simulink model "uncontrolled_simulink"  (R2020b)
settings: Solver=ode15s  StartTime=0.0  StopTime=T  MaxStep=0.01  RelTol=1e-3  EnableMultiTasking=on
values from neighbouring files (symbols this model uses):
  F_ee = zeros(6,1)    [sim_uncontrolled_simulink.m]
  g = [0 -g0 0]'    [sim_uncontrolled_simulink.m]
  info = struct('n_joints', n_joints,                'S', S,                'M_bi', M_bi,                'Inertia', Inertia,                'mass', mass,                'inertial_disp', inertial_disp)    [sim_uncontrolled_simulink.m]
  q_0 = [d0_0 alfa_0 beta_0]    [sim_uncontrolled_simulink.m]
  static_friction = [fs0 fs1 fs2]    [sim_uncontrolled_simulink.m]
  viscous_friction = [fv0 fv1 fv2]    [sim_uncontrolled_simulink.m]
settings Model: Creator=giank  LastModifiedBy=giank
settings DataIOCC: LimitDataPoints=on  MaxDataPoints=10000
settings OptimizationCC: LifeSpan=inf
settings DebuggingCC: AllowSymbolicDim=off  SFUnexpectedBacktrackingDiag=warning  SFNoUnconditionalDefaultTransitionDiag=warning  SFExecutionAtInitializationDiag=none  UnderSpecifiedDimensionMsg=warning  ArithmeticOperatorsInVariantConditions=warning
settings SFSimCC: SimUseLocalCustomCode=off  CustomCodeUndefinedFunction=UseInterfaceOnly
settings RTWCC: RTWUseLocalCustomCode=off
settings CodeAppCC: StateflowObjectComments=on
settings GRTTargetCC: TargetLangStandard=C89/C90 (ANSI)
settings ConfigComp: CovMetricSettings=dw  CovSaveCumulativeToWorkspaceVar=on  CovSaveSingleToWorkspaceVar=on  CovExternalEMLEnable=off  CovSFcnEnable=off
settings SimscapeCC: SimscapeLogType=all  SimscapeLogSimulationStatistics=on  SimscapeLogDataHistory=10000

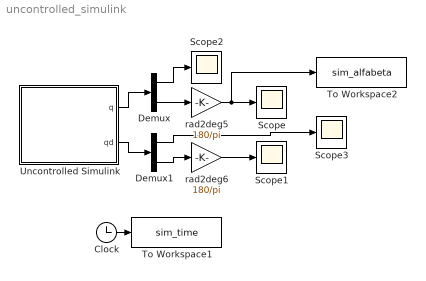
== system uncontrolled_simulink ==
  Clock : Clock
  Demux : Demux  Outputs=[1 2]
  Demux1 : Demux  Outputs=[1 2]
  Scope{,1..3} (4 alike) : Scope
  To Workspace1 : ToWorkspace  VariableName=sim_time  SaveFormat=Timeseries  SampleTime=-1
  To Workspace2 : ToWorkspace  VariableName=sim_alfabeta  SaveFormat=Timeseries  SampleTime=-1
  Uncontrolled Simulink : Subsystem
  rad2deg5 : Gain  Gain=180/pi
  rad2deg6 : Gain  Gain=180/pi
  wires:
  Clock/1 -> To Workspace1/1
  rad2deg6/1 -> Scope1/1
  rad2deg5/1 -> To Workspace2/1, Scope/1
  Demux/2 -> rad2deg5/1
  Uncontrolled Simulink/1(q) -> Demux/1
  Uncontrolled Simulink/2(qd) -> Demux1/1
  Demux1/2 -> rad2deg6/1
  Demux/1 -> Scope2/1
  Demux1/1 -> Scope3/1

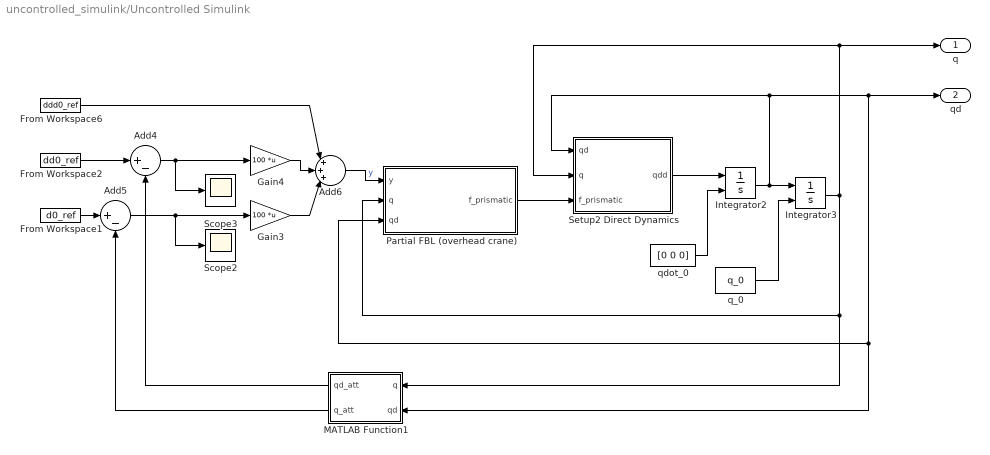
== system uncontrolled_simulink/Uncontrolled Simulink ==
  Add4 : Sum  Inputs=|+-
  Add5 : Sum  Inputs=|+-
  Add6 : Sum  Inputs=|+++|
  From Workspace1 : FromWorkspace  VariableName=d0_ref
  From Workspace2 : FromWorkspace  VariableName=dd0_ref
  From Workspace6 : FromWorkspace  VariableName=ddd0_ref
  Gain3 : Gain  Gain=100  Multiplication=Matrix(K*u)
  Gain4 : Gain  Gain=100  Multiplication=Matrix(K*u)
  Integrator2 : Integrator  InitialConditionSource=external  InitialCondition=[0 0]
  Integrator3 : Integrator  InitialConditionSource=external  InitialCondition=[0 0]
  MATLAB Function1 : MATLAB Function  TreatAsAtomicUnit=on
  Partial FBL (overhead crane) : MATLAB Function  TreatAsAtomicUnit=on
  Scope2 : Scope
  Scope3 : Scope
  Setup2 Direct Dynamics : MATLAB Function  TreatAsAtomicUnit=on
  q_0 : Constant  Value=q_0
  qdot_0 : Constant  Value=[0 0 0]
  q : Outport
  qd : Outport  Port=2
  wires:
  qdot_0/1 -> Integrator2/2
  q_0/1 -> Integrator3/2
  Setup2 Direct Dynamics/1(qdd) -> Integrator2/1
  MATLAB Function1/1(qd_att) -> Add4/2
  Add5/1 -> Gain3/1, Scope2/1
  Add4/1 -> Scope3/1, Gain4/1
  From Workspace2/1 -> Add4/1
  Integrator2/1 -> Integrator3/1, qd/1, MATLAB Function1/2(qd), Partial FBL (overhead crane)/3(qd), Setup2 Direct Dynamics/1(qd)
  Gain3/1 -> Add6/3
  Add6/1 -> Partial FBL (overhead crane)/1(y)  "y"
  Gain4/1 -> Add6/2
  From Workspace6/1 -> Add6/1
  From Workspace1/1 -> Add5/1
  MATLAB Function1/2(q_att) -> Add5/2
  Integrator3/1 -> q/1, Setup2 Direct Dynamics/2(q), MATLAB Function1/1(q), Partial FBL (overhead crane)/2(q)
  Partial FBL (overhead crane)/1(f_prismatic) -> Setup2 Direct Dynamics/3(f_prismatic)

== matlab function uncontrolled_simulink/Uncontrolled Simulink/Partial FBL (overhead crane) ==
  data: y input; q input; f_prismatic output; qd input; g parameter; info parameter; viscous_friction parameter; F_ee parameter; static_friction parameter
function f_prismatic = fcn(y, q, qd, g, info, viscous_friction, F_ee, static_friction)

    % Number of joints
    n_joints = 3;

    % Computation B matrix
    B = zeros(n_joints,n_joints);
    for i=1:n_joints
        fake_acc = zeros(1,n_joints);
        fake_acc(i) = 1;
        B(:,i) = recursive_invdyn_f(q, zeros(1,n_joints), fake_acc, zeros(3,1), info, F_ee);
    end
    
    % Joint friction model
    Fv = diag([viscous_friction(1), viscous_friction(2), viscous_friction(3)]);
    Fs = diag([static_friction(1), static_friction(2), static_friction(3)]);
    friction = Fv*qd + Fs*sign(qd);
    
    % Computation n vector
    n = recursive_invdyn_f(q, qd, zeros(1,n_joints), g, info, F_ee) + friction;

    % Partial Feedback Linearization
    Bm = B(1,1);
    Bmb = B(1,2:3);
    Bbm = B(2:3,1);
    Bb = B(2:3,2:3);
    nb = n(2:3);
    nm = n(1);

    B_tilde = (Bm-Bmb*inv(Bb)*Bbm);
    n_tilde = nm - Bmb*inv(Bb)*nb;

    f_prismatic = B_tilde*y + n_tilde;
    
end

== matlab function uncontrolled_simulink/Uncontrolled Simulink/MATLAB Function1 ==
  data: q input; qd input; qd_att output; q_att output
function [qd_att, q_att] = fcn(q, qd)

qd_att = qd(1);
q_att = q(1);

end

== matlab function uncontrolled_simulink/Uncontrolled Simulink/Setup2 Direct Dynamics ==
  data: qd input; q input; f_prismatic input; qdd output; info parameter; g parameter; viscous_friction parameter; F_ee parameter; static_friction parameter
function qdd = fcn(qd, q, f_prismatic, info, g, viscous_friction, F_ee, static_friction)
    
    % Input
    d0 = q(1);
    alfa = q(2);
    beta = q(3);
    d0_dot = qd(1);
    alfa_dot = qd(2);
    beta_dot = qd(3);
    
    % Number of joints
    n_joints = 3;

    % Computation B matrix
    B = zeros(n_joints,n_joints);
    for i=1:n_joints
        fake_acc = zeros(1,n_joints);
        fake_acc(i) = 1;
        B(:,i) = recursive_invdyn_f(q, zeros(1,n_joints), fake_acc, zeros(3,1), info, F_ee);
    end
    
    % Joint friction model
    Fv = diag([viscous_friction(1), viscous_friction(2), viscous_friction(3)]);
    Fs = diag([static_friction(1), static_friction(2), static_friction(3)]);
    friction = Fv*qd + Fs*sign(qd);
    
    % Computation n vector
    n = recursive_invdyn_f(q, qd, zeros(1,n_joints), g, info, F_ee) + friction;
    
    % Direct dynamics
    G = diag([1 0 0]);
    tau = [f_prismatic; 0; 0];
     
%     tau = [B(1,1)*d0_ddot+n(1); 0; 0];
    
%     qdd = zeros(3,1);
    qdd = (inv(B)*(G*tau-n));

    
    
end
